simulink model "BC_H9"  (R2025a)
settings: Solver=VariableStepAuto  StartTime=0.0  StopTime=2  MaxStep=1e-3  RelTol=1e-3
libraries: simulink_extras x1
settings Model: Creator=Szalay  LastModifiedBy=Szalay

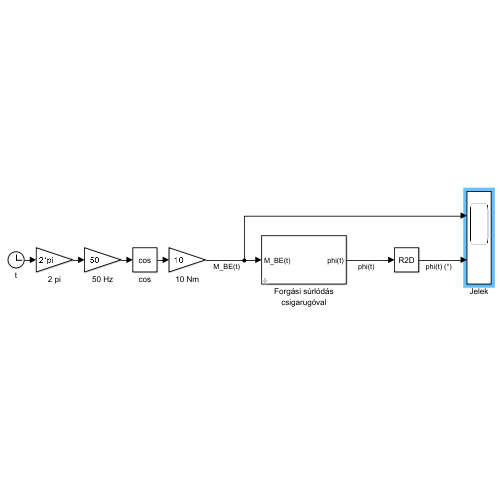
[thumbnail: Simulink's stored preview of the top-level diagram]
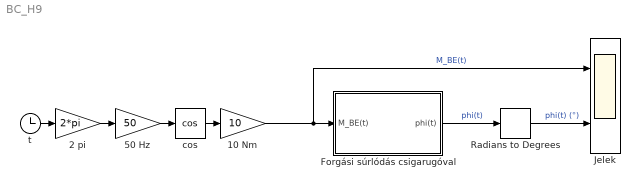
== system BC_H9 ==
  10 Nm : Gain  Gain=10
  2 pi : Gain  Gain=2*pi
  50 Hz : Gain  Gain=50
  Forgási súrlódás csigarugóval : Subsystem  mask(Forgási súrlódás csigarugóval){C=0.5, B=0.1, phi_0=30}
      mask prompts: C "Csavarási rugómerevség (Nm/rad)"; B "Forgási súrlódási együttható (Nms/rad)"; phi_0 "Kezdeti szöghelyzet (°)"
      mask help: Lineáris forgási súrlódásból és lineáris csigarugóból felépülő forgó rendszer.
      mask DialogControl ParameterGroupVar Prompt: Modellparaméterek
      mask DialogControl Container3 Prompt: Kezdeti érték
  Jelek : Scope  NumInputPorts=2
      settings: ActiveDisplayYMinimum=-26.411971296434313  ActiveDisplayYMaximum=55.389626229730247
  Radians to Degrees : simulink_extras/Transformations/Radians to Degrees
  cos : Trigonometry  Operator=cos
  t : Clock
  wires:
  t/1 -> 2 pi/1
  2 pi/1 -> 50 Hz/1
  50 Hz/1 -> cos/1
  cos/1 -> 10 Nm/1
  10 Nm/1 -> Jelek/1, Forgási súrlódás csigarugóval/1(M_BE(t))  "M_BE(t)"
  Forgási súrlódás csigarugóval/1(phi(t)) -> Radians to Degrees/1  "phi(t)"
  Radians to Degrees/1 -> Jelek/2  "phi(t) (°)"

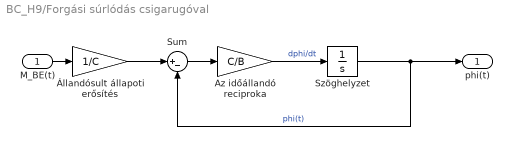
== system BC_H9/Forgási súrlódás csigarugóval ==
  M_BE(t) : Inport
  Az időállandó reciproka : Gain  Gain=C/B
  Sum : Sum  Inputs=|+-
  Szöghelyzet : Integrator  InitialCondition=phi_0 / 180 * pi
  Állandósult állapoti erősítés : Gain  Gain=1/C
  phi(t) : Outport
  wires:
  Szöghelyzet/1 -> Sum/2, phi(t)/1  "phi(t)"
  Sum/1 -> Az időállandó reciproka/1
  M_BE(t)/1 -> Állandósult állapoti erősítés/1
  Az időállandó reciproka/1 -> Szöghelyzet/1  "dphi/dt"
  Állandósult állapoti erősítés/1 -> Sum/1
